simulink model "adithiyhadrivesprojectml"  (R2024a)
settings: Solver=VariableStepAuto  StartTime=0.0  StopTime=0.5  RelTol=1e-3  EnableMultiTasking=on
libraries: spsIGBTDiodeLib x6, spsFourierLib x4, simulink x3, spsGroundLib x2, spsAsynchronousMachineSIUnitsLib x1, spsDCVoltageSourceLib x1, spsIdealSwitchLib x1, spsSawtoothGeneratorLib x1, spsThreePhaseSeriesRLCBranchLib x1, spsThreePhaseVIMeasurementLib x1, spsThreePhaseFaultLib x1, spsVoltageMeasurementLib x1
settings Model: Creator=lenovo 320  LastModifiedBy=Adithiyha R
settings SolverCC: AlgebraicLoopSolver=TrustRegion
settings DataIOCC: InspectSignalLogs=on  ReturnWorkspaceOutputs=off
settings OptimizationCC: LifeSpan=inf
settings DebuggingCC: UnconnectedInputMsg=warning  UnconnectedOutputMsg=warning  UnconnectedLineMsg=warning  SFUnexpectedBacktrackingDiag=warning  SFNoUnconditionalDefaultTransitionDiag=warning  SFExecutionAtInitializationDiag=none  ArithmeticOperatorsInVariantConditions=warning
settings ModelReferenceCC: EnableRefExpFcnMdlSchedulingChecks=on
settings SFSimCC: SimUseLocalCustomCode=off  CustomCodeUndefinedFunction=UseInterfaceOnly
settings RTWCC: RTWUseLocalCustomCode=off  GPUComputeCapability=3.5
settings CodeAppCC: StateflowObjectComments=on
settings GRTTargetCC: TargetLangStandard=C89/C90 (ANSI)
settings ConfigComp: CovMetricSettings=dw  CovSaveCumulativeToWorkspaceVar=on  CovSaveSingleToWorkspaceVar=on  CovExternalEMLEnable=off
settings SimscapeCC: SimscapeNormalizeSystem=off

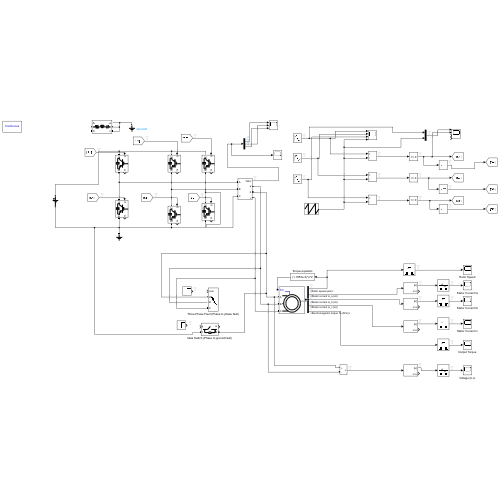
[thumbnail: Simulink's stored preview of the top-level diagram]
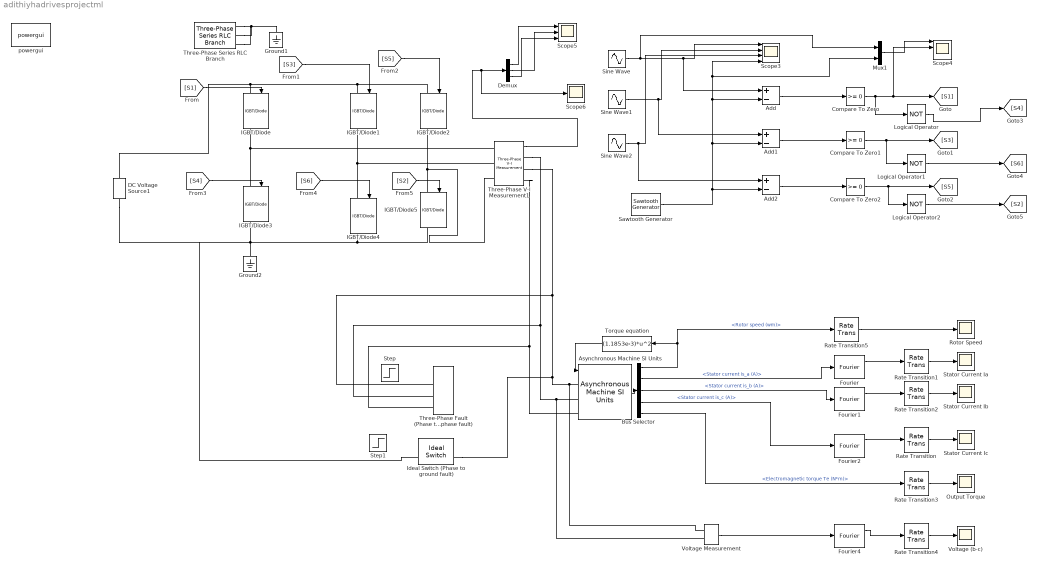
== system adithiyhadrivesprojectml ==
  Add : Sum  Inputs=+-
  Add1 : Sum  Inputs=+-
  Add2 : Sum  Inputs=+-
  Asynchronous Machine SI Units : spsAsynchronousMachineSIUnitsLib/Asynchronous Machine SI Units  RotorType=Squirrel-cage  PresetModel="15:  5.4 HP (4KW)   400 V  50Hz 1430 RPM"  MechanicalLoad=Torque Tm  ShowDetailedParameters=on  ReferenceFrame=Rotor  Units=SI  MeasurementBus=off  NominalParameters=[4000 400 50]  VoltageRatio=1  Stator=[1.405 0.005839]  Rotor=[1.395 0.005839]  Cage1=[0.4155 0.002066]  Cage2=[0.4168 0.0003495]  Lm=0.1722  Mechanical=[0.0131 0.002985 2]  PolePairs=2  InitialConditions=[0 0 0 0 0 0 0 0]  SimulateSaturation=off  Saturation=[14.03593122, 27.81365428, 53.79336849, 72.68890987, 97.98006896, 148.6815601, 215.7428561, 302.9841135, 428.7778367 ; 230, 322, 414, 460, 506, 552, 598, 644, 690]  LoadFlowParameters=1492000  TsPowergui=0  TsBlock=-1  IterativeModel=Trapezoidal non iterative  IterativeDiscreteModel=Trapezoidal non iterative  Pmec=1.492e+006
  Bus Selector : BusSelector  OutputSignals=Mechanical.Rotor speed (wm),Stator measurements.Stator current is_a (A),Stator measurements.Stator current is_b (A),Stator measurements.Stator current is_c (A),Mechanical.Electromagnetic torque Te (N*m)
  Compare To Zero : simulink/Logic and Bit Operations/Compare To Zero  relop=>=  OutDataTypeStr=boolean
  Compare To Zero1 : simulink/Logic and Bit Operations/Compare To Zero  relop=>=  OutDataTypeStr=boolean
  Compare To Zero2 : simulink/Logic and Bit Operations/Compare To Zero  relop=>=  OutDataTypeStr=boolean
  DC Voltage Source1 : spsDCVoltageSourceLib/DC Voltage Source  Amplitude=548.5  Measurements=Voltage
  Demux : Demux  Outputs=3
  Fourier{,1..2,4} (4 alike) : spsFourierLib/Fourier  Freq=50  n=1  InInit=[0, 0]  Ts=0
  Ground1 : spsGroundLib/Ground  LConnTagsString=a
  Ground2 : spsGroundLib/Ground  LConnTagsString=a
  IGBT/Diode{,1..5} (6 alike) : spsIGBTDiodeLib/IGBT//Diode  Ron=1e-3  Rs=1e5  Cs=inf  Measurements=on
  Ideal Switch (Phase to ground fault) : spsIdealSwitchLib/Ideal Switch  Ron=0.001  Lon=0  IC=0  Rs=1e6  Cs=inf  Measurements=on
  Logical Operator : Logic  Operator=NOT  AllPortsSameDT=off  OutDataTypeStr=boolean
  Logical Operator1 : Logic  Operator=NOT  AllPortsSameDT=off  OutDataTypeStr=boolean
  Logical Operator2 : Logic  Operator=NOT  AllPortsSameDT=off  OutDataTypeStr=boolean
  Mux1 : Mux  Inputs=2
  Output Torque : Scope
  Rate Transition{,1..5} (6 alike) : RateTransition  OutPortSampleTimeMultiple=500  OutPortSampleTime=0.0005
  Rotor Speed : Scope
  Sawtooth Generator : spsSawtoothGeneratorLib/Sawtooth Generator  Freq=1e3  Phase=180  Ts=0
  Scope3 : Scope  NumInputPorts=4
  Scope4 : Scope  NumInputPorts=4
  Scope5 : Scope  NumInputPorts=3
  Scope6 : Scope
  Sine Wave : Sin  Frequency=2*pi*50  SampleTime=0
  Sine Wave1 : Sin  Frequency=2*pi*50  Phase=+2*pi/3  SampleTime=0
  Sine Wave2 : Sin  Frequency=2*pi*50  Phase=-2*pi/3  SampleTime=0
  Stator Current Ia : Scope
  Stator Current Ib : Scope
  Stator Current Ic : Scope
  Step : Step  Time=0.1  SampleTime=10e-6
  Step1 : Step  Time=0.1  SampleTime=10e-6
  Three-Phase Series RLC Branch : spsThreePhaseSeriesRLCBranchLib/Three-Phase Series RLC Branch  LConnTagsString=A|B|C  RConnTagsString=A|B|C  BranchType=RLC  Resistance=1  Inductance=1e-3  Capacitance=1e-6  Measurements=None
  Three-Phase V-I Measurement1 : spsThreePhaseVIMeasurementLib/Three-Phase V-I Measurement  VoltageMeasurement=phase-to-phase  SetLabelV=off  LabelV=Vabc  Vpu=off  VpuLL=off  CurrentMeasurement=no  SetLabelI=off  LabelI=Iabc  Ipu=off  Pbase=100e6  Vbase=500e3  OutputType=Complex  PhasorSimulation=off  PSBequivalent=0
  Three-Phase Fault (Phase to phase fault) : spsThreePhaseFaultLib/Three-Phase Fault  InitialStates=0  FaultA=on  FaultB=on  FaultC=off  GroundFault=off  SwitchTimes="[1/60  5/60]"  External=on  SwitchStatus=NaN  FaultResistance=0.001  GroundResistance=0.001  SnubberResistance=1e6  SnubberCapacitance=inf  Measurements=None
  Torque equation : Fcn  Expr=(1.1853e-3)*u^2
  Voltage (b-c) : Scope
  Voltage Measurement : spsVoltageMeasurementLib/Voltage Measurement  PhasorSimulation=off  OutputType=Complex  PSBequivalent=0
  powergui : spspowerguiLib/powergui  Priority=1  SimulationMode=Continuous  SampleTime=50e-6  frequency=60  Iterations=50  frequencyindice=0  Pbase=100e6  ErrMax=1e-4  UnitsV=kV  UnitsW=MW  buscounter=0  FunctionMessages=off  echomessages=off  EnableUseOfTLC=off  CurrentSourceSwitches=off  DisableSnubberDevices=off  DisableRonSwitches=off  DisableVfSwitches=off  DisplayEquations=off  AutomaticDiscreteSolvers=off  SolverType=Tustin/Backward Euler (TBE)  Interpol=off  ExternalGateDelay=off  methode=off  Ts=100  x0status=blocks  SPID=off  SwTol=0  HookPort=off  NonlinearTolerance=1e-4  nMaxIteration=100  ContinueOnMaxIteration=off  RestoreLinks=warning  ResistiveCurrentMeasurement=off  Frange=[0:2:500]  Ylog=off  Xlog=on  ShowGrid=off  save=off  variable=ZData  structure=0  ZoomFFT=off  StartTime=0.0  cycles=1  DisplayStyle=1  fundamental=60  FreqAxis=off  MaxFrequency=1000  frequencyindicesteady=1  RmsSteady=1  display=off
  wires:
  Sine Wave/1 -> Mux1/1, Add/1, Scope3/1
  Sine Wave1/1 -> Add1/1, Scope3/2
  Sine Wave2/1 -> Add2/1, Scope3/3
  Sawtooth Generator/1 -> Add2/2, Add1/2, Add/2, Mux1/2, Scope3/4
  Add/1 -> Compare To Zero/1
  Add1/1 -> Compare To Zero1/1
  Add2/1 -> Compare To Zero2/1
  Mux1/1 -> Scope4/1
  Compare To Zero/1 -> Logical Operator/1, [S1], Scope4/2
  Compare To Zero1/1 -> Logical Operator1/1, [S3]
  Compare To Zero2/1 -> Logical Operator2/1, [S5]
  Logical Operator/1 -> [S4]
  Logical Operator1/1 -> [S6]
  Logical Operator2/1 -> [S2]
  [S1] -> IGBT/Diode/1
  [S3] -> IGBT/Diode1/1
  [S5] -> IGBT/Diode2/1
  [S4] -> IGBT/Diode3/1
  [S6] -> IGBT/Diode4/1
  [S2] -> IGBT/Diode5/1
  Three-Phase V-I Measurement1/1 -> Scope6/1, Demux/1
  Demux/1 -> Scope5/1
  Demux/2 -> Scope5/2
  Demux/3 -> Scope5/3
  Asynchronous Machine SI Units/1 -> Bus Selector/1
  Bus Selector/2 -> Fourier/1  "<Stator current is_a (A)>"
  Bus Selector/4 -> Fourier2/1  "<Stator current is_c (A)>"
  Bus Selector/1 -> Rate Transition5/1, Torque equation/1  "<Rotor speed (wm)>"
  Torque equation/1 -> Asynchronous Machine SI Units/1
  Voltage Measurement/1 -> Fourier4/1
  Fourier2/1 -> Rate Transition/1
  Bus Selector/3 -> Fourier1/1  "<Stator current is_b (A)>"
  Rate Transition/1 -> Stator Current Ic/1
  Fourier/1 -> Rate Transition1/1
  Rate Transition1/1 -> Stator Current Ia/1
  Fourier1/1 -> Rate Transition2/1
  Rate Transition2/1 -> Stator Current Ib/1
  Bus Selector/5 -> Rate Transition3/1  "<Electromagnetic torque Te (N*m)>"
  Rate Transition3/1 -> Output Torque/1
  Fourier4/1 -> Rate Transition4/1
  Rate Transition4/1 -> Voltage (b-c)/1
  Rate Transition5/1 -> Rotor Speed/1
  connections:
  Three-Phase V-I Measurement1/LConn1 -- IGBT/Diode/RConn1 -- IGBT/Diode3/LConn1
  Three-Phase V-I Measurement1/LConn2 -- IGBT/Diode1/RConn1 -- IGBT/Diode4/LConn1
  IGBT/Diode5/LConn1 -- IGBT/Diode2/RConn1 -- Three-Phase V-I Measurement1/LConn3
  Three-Phase Series RLC Branch/RConn1 -- Three-Phase Series RLC Branch/RConn3 -- Three-Phase Series RLC Branch/RConn2 -- Ground1/LConn1
  IGBT/Diode/LConn1 -- DC Voltage Source1/RConn1 -- IGBT/Diode2/LConn1 -- IGBT/Diode1/LConn1
  IGBT/Diode4/RConn1 -- IGBT/Diode5/RConn1 -- Ground2/LConn1 -- Ideal Switch (Phase to ground fault)/LConn1 -- DC Voltage Source1/LConn1 -- IGBT/Diode3/RConn1
  Three-Phase V-I Measurement1/RConn3 -- Asynchronous Machine SI Units/LConn3 -- Three-Phase Fault (Phase to phase fault)/LConn3
  Three-Phase V-I Measurement1/RConn2 -- Ideal Switch (Phase to ground fault)/RConn1 -- Voltage Measurement/LConn1 -- Asynchronous Machine SI Units/LConn1 -- Three-Phase Fault (Phase to phase fault)/LConn1
  Three-Phase V-I Measurement1/RConn1 -- Voltage Measurement/LConn2 -- Asynchronous Machine SI Units/LConn2 -- Three-Phase Fault (Phase to phase fault)/LConn2
